simulink subsystem "circle_generator"  (R2019b)
settings: Solver=VariableStepAuto  StartTime=0.0  StopTime=10.0  RelTol=1e-3
libraries: quarc_library x2, SignalEditorBlockLib x1
settings Model: Creator=icpmoles  LastModifiedBy=icpmoles

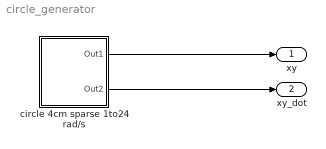
== system circle_generator ==
  circle 4cm sparse 1to24 rad/s : Subsystem
  xy : Outport
  xy_dot : Outport  Port=2
  wires:
  circle 4cm sparse 1to24 rad/s/1(Out1) -> xy/1
  circle 4cm sparse 1to24 rad/s/2(Out2) -> xy_dot/1

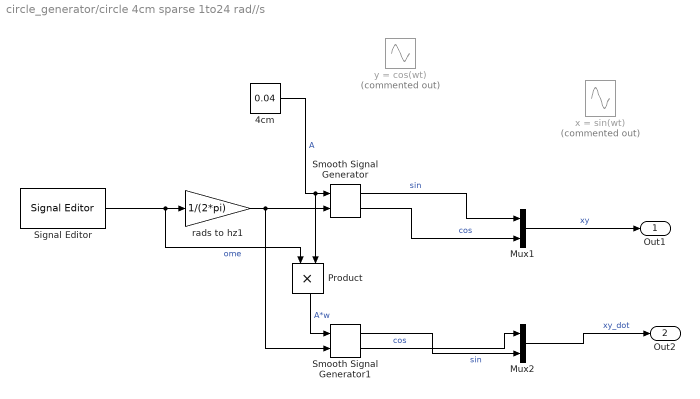
== system circle_generator/circle 4cm sparse 1to24 rad//s ==
  4cm : Constant  Value=0.04
  Mux1 : Mux  Inputs=2
  Mux2 : Mux  Inputs=2
  Product : Product
  Signal Editor : SignalEditorBlockLib/Signal Editor  FileName=circle_omega.mat  ActiveScenario=circle  ActiveSignal=wxy  IsBus=off  OutputBusObjectStr=Bus: BusObject  SampleTime=0  Interpolate=off  ZeroCross=off  OutputAfterFinalValue=Setting to zero  Unit=inherit  PreserveSignalName=on
      settings: SourceProductName=Simulink
  Smooth Signal Generator : quarc_library/Sources/Signals/Smooth Signal Generator  signal_type=Sine  source=External (input ports)  amplitude=1  frequency=1  initial_phase=0  sample_time=qc_get_step_size  output_cos=on
      settings: SourceProductName=QUARC Targets
  Smooth Signal Generator1 : quarc_library/Sources/Signals/Smooth Signal Generator  signal_type=Sine  source=External (input ports)  amplitude=1  frequency=1  initial_phase=0  sample_time=qc_get_step_size  output_cos=on
      settings: SourceProductName=QUARC Targets
  rads to hz1 : Gain  Gain=1/(2*pi)
  x = sin(wt) : Sin  Commented=on  Amplitude=0.04  Frequency=2  SampleTime=0
  y = cos(wt) : Sin  Commented=on  Amplitude=0.04  Frequency=2  Phase=pi/2  SampleTime=0
  Out1 : Outport
  Out2 : Outport  Port=2
  wires:
  Smooth Signal Generator/1 -> Mux1/1  "sin"
  Smooth Signal Generator/2 -> Mux1/2  "cos"
  Mux1/1 -> Out1/1  "xy"
  Signal Editor/1 -> Product/1, rads to hz1/1  "ome"
  rads to hz1/1 -> Smooth Signal Generator1/2, Smooth Signal Generator/2
  4cm/1 -> Product/2, Smooth Signal Generator/1  "A"
  Mux2/1 -> Out2/1  "xy_dot"
  Smooth Signal Generator1/1 -> Mux2/2  "sin"
  Smooth Signal Generator1/2 -> Mux2/1  "cos"
  Product/1 -> Smooth Signal Generator1/1  "A*w"
